simulink model "simu_Ex1"  (R2019b)
settings: Solver=VariableStepAuto  StartTime=0.0  StopTime=10.0  RelTol=1e-3
undefined symbols (not defined in the file): A, B, C, G, J, L
settings Model: Creator=Alex  LastModifiedBy=huojiaxi
settings DataIOCC: ReturnWorkspaceOutputs=off
settings DebuggingCC: ArithmeticOperatorsInVariantConditions=warning
settings SFSimCC: SimUseLocalCustomCode=off  CustomCodeUndefinedFunction=UseInterfaceOnly
settings RTWCC: RTWUseLocalCustomCode=off

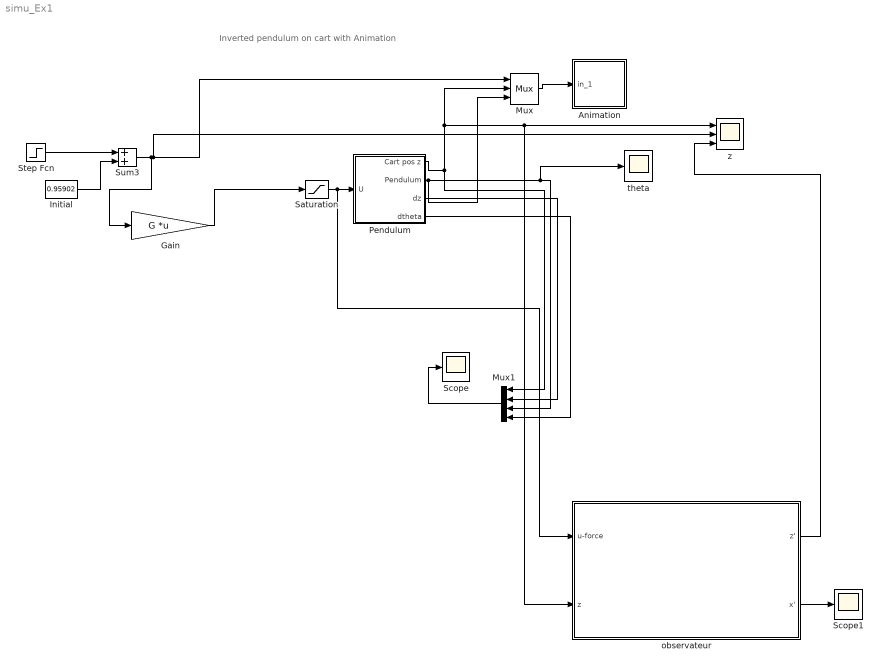
== system simu_Ex1 ==
  note: Inverted pendulum on cart with Animation
  Animation : Subsystem  mask(Pendulum plot){RefBlock=Initial}
      mask prompts: RefBlock "DC reference signal block name:"
      mask help: Pendulum plot
      mask Help: Pendulum animation function using Handle graphics.
      mask Display: plot([-10 10],[0 0],[-2 -2 2 2],[0 1 1 0],[0 3],[1 5])
  Gain : Gain  Gain=G  Multiplication=Matrix(K*u) (u vector)
  Initial : Constant  Value=0.95902
  Mux : Mux  Inputs=3
  Mux1 : Mux
  Pendulum : Subsystem  mask(Inverted pendulum on cart){Mcart=0.455, m=0.21, l=0.61/2, g=9.8}
      mask prompts: Mcart "Mass of cart (kg):"; m "Mass of pendulum (kg):"; l "Distance to pendulum center of mass(m):"; g "Acceleration of gravity (m/s^2):"
      mask help: Unmask and double-click to see dynamics
      mask Help: Nonlinear dynamics of inverted pendulum on cart.
  Saturation : Saturate  UpperLimit=10  LowerLimit=-10
  Scope : Scope
  Scope1 : Scope
  Step Fcn : Step  Time=0  After=10  SampleTime=0
  Sum3 : Sum  SaturateOnIntegerOverflow=on  InputSameDT=on  OutDataTypeStr=Inherit: Same as first input
  "observateur " : Subsystem
  theta : Scope
  z : Scope  NumInputPorts=3
  wires:
  Mux/1 -> Animation/1(in_1)
  Initial/1 -> Sum3/2
  Pendulum/1(Cart pos z) -> Mux1/1, "observateur "/2(z), z/1, Mux/2
  Saturation/1 -> "observateur "/1(u-force), Pendulum/1(U)
  Pendulum/3(dz) -> Mux1/2
  Pendulum/2(Pendulum) -> theta/1, Mux1/3, Mux/3
  Pendulum/4("dtheta ") -> Mux1/4
  Step Fcn/1 -> Sum3/1
  Sum3/1 -> Gain/1, z/2, Mux/1
  Gain/1 -> Saturation/1
  "observateur "/1(z') -> z/3
  Mux1/1 -> Scope/1
  "observateur "/2(x') -> Scope1/1

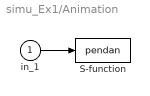
== system simu_Ex1/Animation ==
  in_1 : Inport
  S-function : S-Function  FunctionName=pendan  Parameters=RefBlock  SFunctionDeploymentMode=off  EnableBusSupport=off
      settings: DeleteFcn=pendan([],[],[],'DeleteBlock');
  wires:
  in_1/1 -> S-function/1

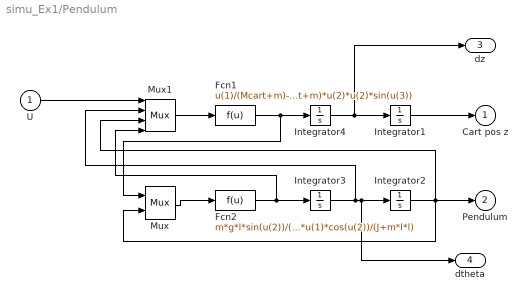
== system simu_Ex1/Pendulum ==
  U : Inport
  Fcn1 : Fcn  Expr=u(1)/(Mcart+m)-m*l/(Mcart+m)*u(4)*cos(u(3))+m*l/(Mcart+m)*u(2)*u(2)*sin(u(3))
  Fcn2 : Fcn  Expr=m*g*l*sin(u(2))/(J+m*l*l)-m*l*u(1)*cos(u(2))/(J+m*l*l)
  Integrator1 : Integrator
  Integrator2 : Integrator  InitialCondition=0.01
  Integrator3 : Integrator
  Integrator4 : Integrator
  Mux : Mux  Inputs=2
  Mux1 : Mux
  Cart pos z : Outport  InitialOutput=0  VectorParamsAs1DForOutWhenUnconnected=off
  Pendulum : Outport  Port=2  InitialOutput=0  VectorParamsAs1DForOutWhenUnconnected=off
  dz : Outport  Port=3  VectorParamsAs1DForOutWhenUnconnected=off
  "dtheta " : Outport  Port=4  VectorParamsAs1DForOutWhenUnconnected=off
  wires:
  Integrator1/1 -> Cart pos z/1
  Fcn2/1 -> Mux1/4, Integrator3/1
  Mux/1 -> Fcn2/1
  Mux1/1 -> Fcn1/1
  Fcn1/1 -> Mux/1, Integrator4/1
  Integrator4/1 -> dz/1, Integrator1/1
  U/1 -> Mux1/1
  Integrator3/1 -> "dtheta "/1, Integrator2/1, Mux1/2
  Integrator2/1 -> Mux/2, Pendulum/1, Mux1/3

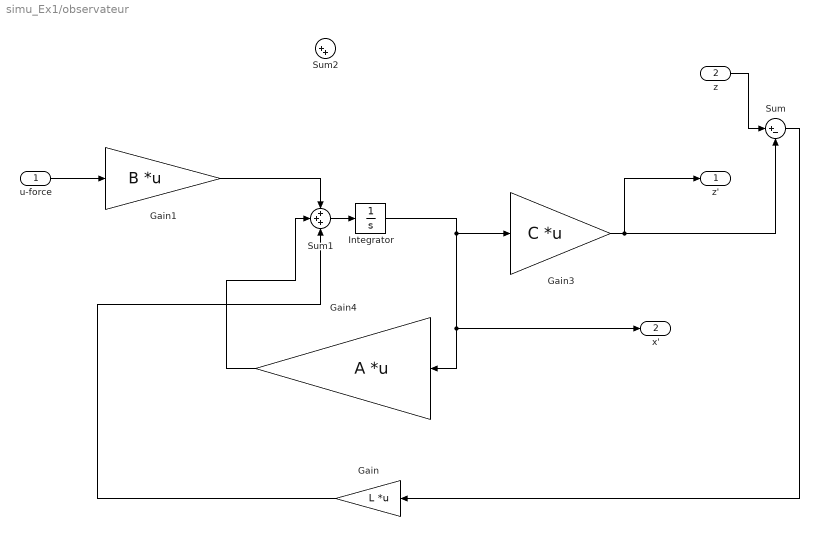
== system simu_Ex1/observateur  ==
  u-force : Inport
  z : Inport  Port=2
  Gain : Gain  Gain=L  Multiplication=Matrix(K*u) (u vector)
  Gain1 : Gain  Gain=B  Multiplication=Matrix(K*u) (u vector)
  Gain3 : Gain  Gain=C  Multiplication=Matrix(K*u) (u vector)
  Gain4 : Gain  Gain=A  Multiplication=Matrix(K*u) (u vector)
  Integrator : Integrator
  Sum : Sum  Inputs=|+-
  Sum1 : Sum  Inputs=+++
  Sum2 : Sum  Inputs=|++
  z' : Outport  VectorParamsAs1DForOutWhenUnconnected=off
  x' : Outport  Port=2  VectorParamsAs1DForOutWhenUnconnected=off
  wires:
  Gain4/1 -> Sum1/2
  Gain1/1 -> Sum1/1
  Sum1/1 -> Integrator/1
  Integrator/1 -> x'/1, Gain4/1, Gain3/1
  Gain3/1 -> Sum/2, z'/1
  z/1 -> Sum/1
  Sum/1 -> Gain/1
  Gain/1 -> Sum1/3
  u-force/1 -> Gain1/1
